simulink model "pendule_inv_etu5"  (R2021a)
settings: Solver=VariableStepAuto  StartTime=0.0  StopTime=10.0  RelTol=1e-3
undefined symbols (not defined in the file): g, K, l, ue, x0, xe
settings Model: Creator=yyounes  LastModifiedBy=yyounes

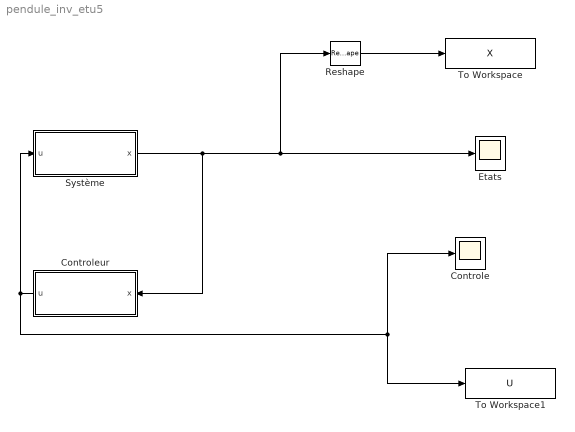
== system pendule_inv_etu5 ==
  Controle : Scope
  Controleur : Subsystem
  Etats : Scope
  Reshape : Reshape
  Système : Subsystem
  To Workspace : ToWorkspace  VariableName=X  SaveFormat=Timeseries  SampleTime=-1
  To Workspace1 : ToWorkspace  VariableName=U  SaveFormat=Timeseries  SampleTime=-1
  wires:
  Controleur/1(u) -> Controle/1, To Workspace1/1, Système/1(u)
  Système/1(x) -> Etats/1, Reshape/1, Controleur/1(x)
  Reshape/1 -> To Workspace/1

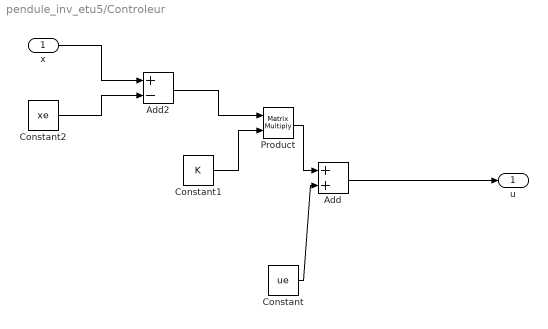
== system pendule_inv_etu5/Controleur ==
  x : Inport
  Add : Sum
  Add2 : Sum  Inputs=+-
  Constant : Constant  Value=ue
  Constant1 : Constant  Value=K
  Constant2 : Constant  Value=xe
  Product : Product  Multiplication=Matrix(*)
  u : Outport
  wires:
  Add/1 -> u/1
  Constant2/1 -> Add2/2
  x/1 -> Add2/1
  Constant1/1 -> Product/2
  Add2/1 -> Product/1
  Product/1 -> Add/1
  Constant/1 -> Add/2

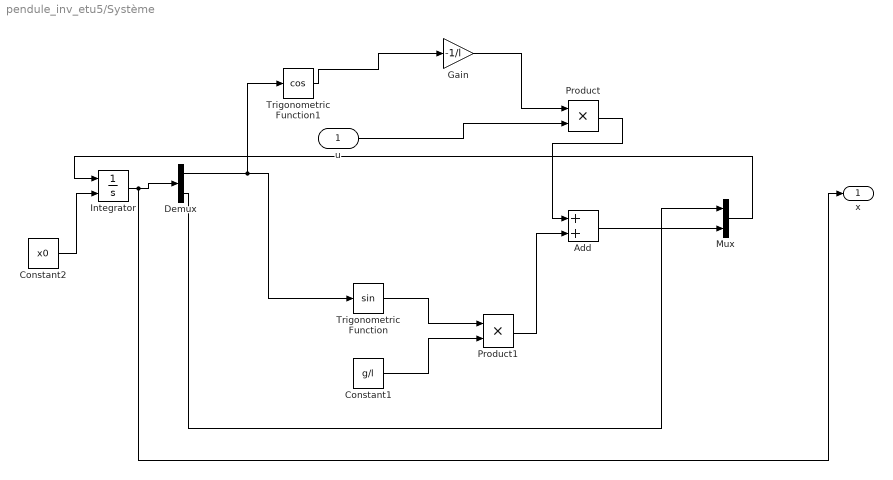
== system pendule_inv_etu5/Système ==
  u : Inport
  Add : Sum
  Constant1 : Constant  Value=g/l
  Constant2 : Constant  Value=x0
  Demux : Demux  Outputs=2
  Gain : Gain  Gain=-1/l
  Integrator : Integrator  InitialConditionSource=external
  Mux : Mux  Inputs=2
  Product : Product
  Product1 : Product
  Trigonometric Function : Trigonometry
  Trigonometric Function1 : Trigonometry  Operator=cos
  x : Outport
  wires:
  Trigonometric Function1/1 -> Gain/1
  Demux/1 -> Trigonometric Function/1, Trigonometric Function1/1
  Constant1/1 -> Product1/2
  Trigonometric Function/1 -> Product1/1
  Product1/1 -> Add/2
  Add/1 -> Mux/2
  Demux/2 -> Mux/1
  Integrator/1 -> x/1, Demux/1
  Mux/1 -> Integrator/1
  Constant2/1 -> Integrator/2
  Gain/1 -> Product/1
  Product/1 -> Add/1
  u/1 -> Product/2
